simulink model "MFC_SISO"  (R2026a)
settings: Solver=VariableStepAuto  StopTime=t_simu
values from neighbouring files (symbols this model uses):
  a = 2.5348    [slexAircraftPitchControlData.mat]
  b = 64.13    [slexAircraftPitchControlData.mat]
  Md = -6.8847    [slexAircraftPitchControlData.mat]
  Mq = -0.6571    [slexAircraftPitchControlData.mat]
  Mw = -0.00592    [slexAircraftPitchControlData.mat]
  Swg = 3    [slexAircraftPitchControlData.mat]
  Uo = 689.4    [slexAircraftPitchControlData.mat]
  Vto = 690.4    [slexAircraftPitchControlData.mat]
  Zd = -63.9979    [slexAircraftPitchControlData.mat]
  Zw = -0.6385    [slexAircraftPitchControlData.mat]
undefined symbols (not defined in the file or in its folder): Ts
libraries: aerolibactuator x2, simulink x1
settings Model: Creator=devinbellll  LastModifiedBy=devinbellll

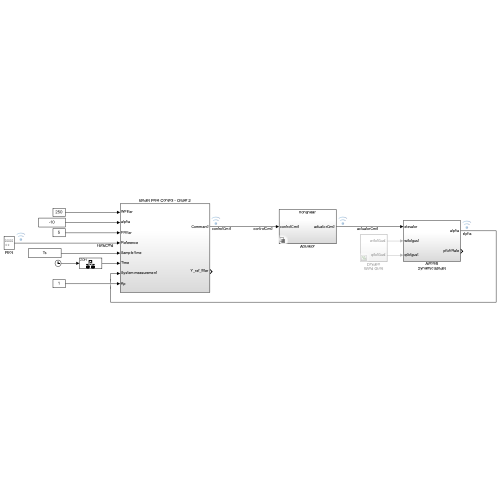
[thumbnail: Simulink's stored preview of the top-level diagram]
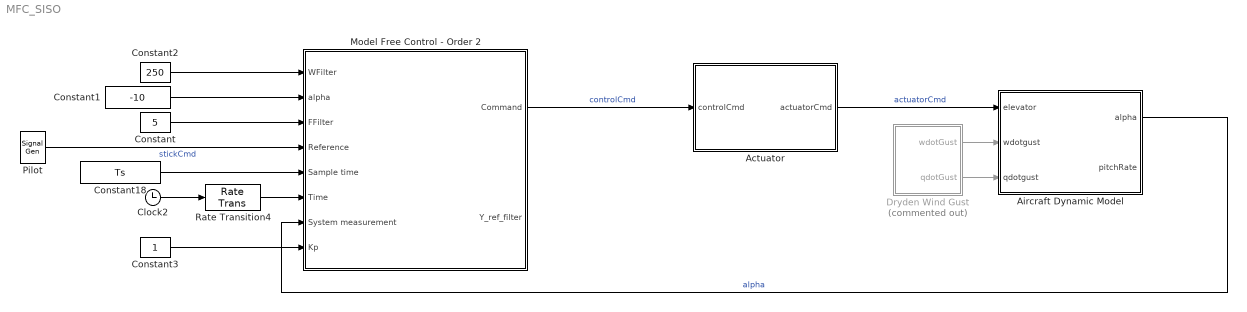
== system MFC_SISO ==
  Actuator : Subsystem  Variant=on  VariantControlMode=label  LabelModeActiveChoice=NonlinearActuator
  Aircraft Dynamic Model : Subsystem
  Clock2 : Clock
  Constant : Constant  Value=5
  Constant1 : Constant  Value=-10
  Constant18 : Constant  Value=Ts  SampleTime=-1
  Constant2 : Constant  Value=250
  Constant3 : Constant
  Dryden Wind Gust : Subsystem  Commented=on
  Model Free Control - Order 2 : Subsystem
  Pilot : SignalGenerator  WaveForm=square  Frequency=.1
  Rate Transition4 : RateTransition  OutPortSampleTime=Ts
  wires:
  Constant3/1 -> Model Free Control - Order 2/8(Kp)
  Clock2/1 -> Rate Transition4/1
  Rate Transition4/1 -> Model Free Control - Order 2/6(Time)
  Constant18/1 -> Model Free Control - Order 2/5(Sample time)
  Constant/1 -> Model Free Control - Order 2/3(FFilter)
  Pilot/1 -> Model Free Control - Order 2/4(Reference)  "stickCmd"
  Constant2/1 -> Model Free Control - Order 2/1(WFilter)
  Constant1/1 -> Model Free Control - Order 2/2(alpha)
  Model Free Control - Order 2/1(Command) -> Actuator/1(controlCmd)  "controlCmd"
  Dryden Wind Gust/1(wdotGust) -> Aircraft Dynamic Model/2(wdotgust)
  Actuator/1(actuatorCmd) -> Aircraft Dynamic Model/1(elevator)  "actuatorCmd"
  Dryden Wind Gust/2(qdotGust) -> Aircraft Dynamic Model/3(qdotgust)
  Aircraft Dynamic Model/1(alpha) -> Model Free Control - Order 2/7(System measurement)  "alpha"

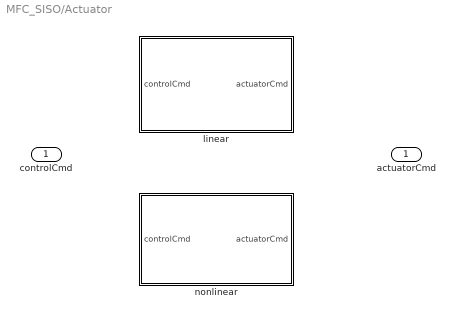
== system MFC_SISO/Actuator ==
  controlCmd : Inport
  linear : Subsystem  VariantControl=LinearActuator
  nonlinear : Subsystem  VariantControl=NonlinearActuator
  actuatorCmd : Outport  InitialOutput=0  VectorParamsAs1DForOutWhenUnconnected=off

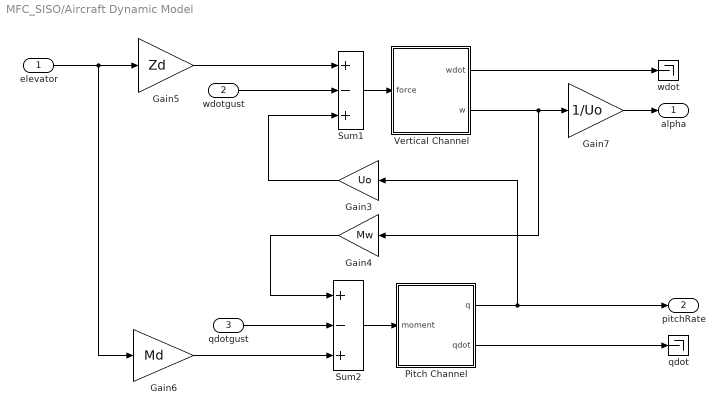
== system MFC_SISO/Aircraft Dynamic Model ==
  elevator : Inport
  wdotgust : Inport  Port=2
  qdotgust : Inport  Port=3
  Gain3 : Gain  Gain=Uo  SaturateOnIntegerOverflow=on  OutDataTypeStr=Inherit: Same as input  ParamDataTypeStr=Inherit: Same as input
  Gain4 : Gain  Gain=Mw  SaturateOnIntegerOverflow=on  OutDataTypeStr=Inherit: Same as input  ParamDataTypeStr=Inherit: Same as input
  Gain5 : Gain  Gain=Zd  SaturateOnIntegerOverflow=on  OutDataTypeStr=Inherit: Same as input  ParamDataTypeStr=Inherit: Same as input
  Gain6 : Gain  Gain=Md  SaturateOnIntegerOverflow=on  OutDataTypeStr=Inherit: Same as input  ParamDataTypeStr=Inherit: Same as input
  Gain7 : Gain  Gain=1/Uo  SaturateOnIntegerOverflow=on  OutDataTypeStr=Inherit: Same as input  ParamDataTypeStr=Inherit: Same as input
  Pitch Channel : Subsystem
  Sum1 : Sum  Inputs=+-+  InputSameDT=on  SaturateOnIntegerOverflow=on  OutDataTypeStr=Inherit: Same as first input
  Sum2 : Sum  Inputs=+-+  InputSameDT=on  SaturateOnIntegerOverflow=on  OutDataTypeStr=Inherit: Same as first input
  Vertical Channel : Subsystem
  qdot : Terminator
  wdot : Terminator
  alpha : Outport
  pitchRate : Outport  Port=2
  wires:
  Pitch Channel/1(q) -> Gain3/1, pitchRate/1
  Vertical Channel/2(w) -> Gain7/1, Gain4/1
  Sum1/1 -> Vertical Channel/1(force)
  Gain6/1 -> Sum2/3
  Gain5/1 -> Sum1/1
  qdotgust/1 -> Sum2/2
  Sum2/1 -> Pitch Channel/1(moment)
  wdotgust/1 -> Sum1/2
  elevator/1 -> Gain6/1, Gain5/1
  Gain7/1 -> alpha/1
  Gain3/1 -> Sum1/3
  Gain4/1 -> Sum2/1
  Vertical Channel/1(wdot) -> wdot/1
  Pitch Channel/2(qdot) -> qdot/1

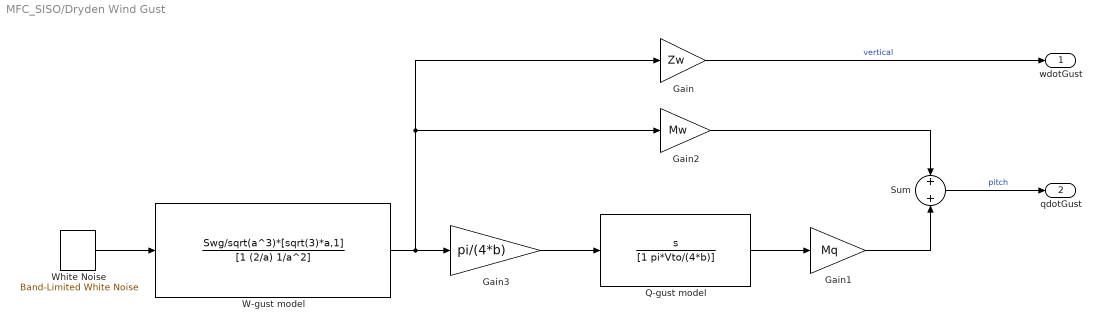
== system MFC_SISO/Dryden Wind Gust ==
  Gain : Gain  Gain=Zw  SaturateOnIntegerOverflow=on  OutDataTypeStr=Inherit: Same as input  ParamDataTypeStr=Inherit: Same as input
  Gain1 : Gain  Gain=Mq  SaturateOnIntegerOverflow=on  OutDataTypeStr=Inherit: Same as input  ParamDataTypeStr=Inherit: Same as input
  Gain2 : Gain  Gain=Mw  SaturateOnIntegerOverflow=on  OutDataTypeStr=Inherit: Same as input  ParamDataTypeStr=Inherit: Same as input
  Gain3 : Gain  Gain=pi/(4*b)  SaturateOnIntegerOverflow=on  OutDataTypeStr=Inherit: Same as input  ParamDataTypeStr=Inherit: Same as input
  Q-gust model : TransferFcn  Numerator=[1 0]  Denominator=[1 pi*Vto/(4*b)]
  Sum : Sum  InputSameDT=on  SaturateOnIntegerOverflow=on  OutDataTypeStr=Inherit: Same as first input
  W-gust model : TransferFcn  Numerator=Swg/sqrt(a^3)*[sqrt(3)*a,1]  Denominator=[1 (2/a) 1/a^2]
  White Noise : simulink/Sources/Band-Limited White Noise  Cov=10  Ts=0.01  seed=23341
  wdotGust : Outport  VectorParamsAs1DForOutWhenUnconnected=off
  qdotGust : Outport  Port=2  VectorParamsAs1DForOutWhenUnconnected=off
  wires:
  Gain/1 -> wdotGust/1  "vertical"
  White Noise/1 -> W-gust model/1
  Gain3/1 -> Q-gust model/1
  Sum/1 -> qdotGust/1  "pitch"
  Gain2/1 -> Sum/1
  Q-gust model/1 -> Gain1/1
  W-gust model/1 -> Gain/1, Gain2/1, Gain3/1
  Gain1/1 -> Sum/2

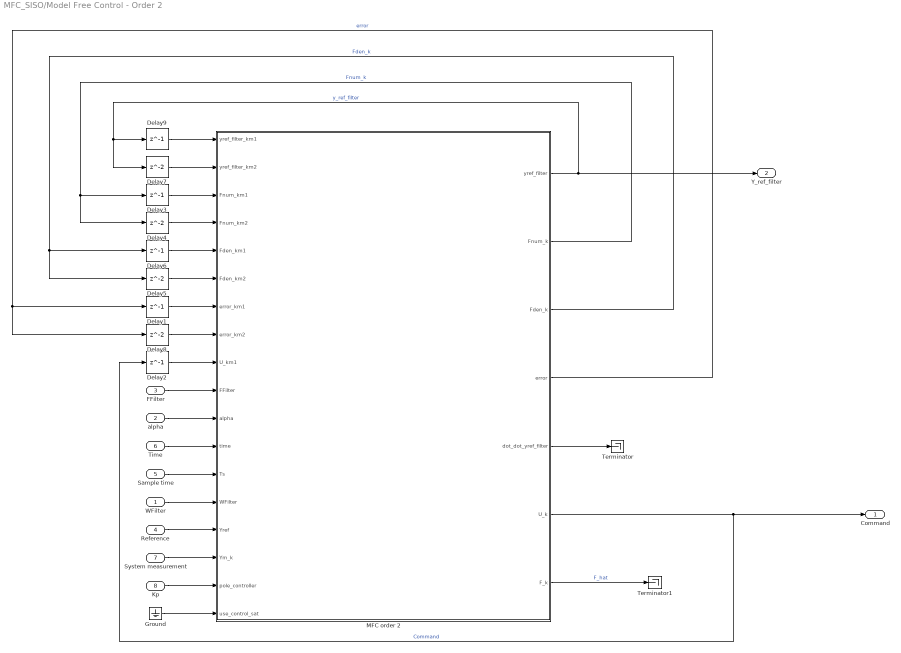
== system MFC_SISO/Model Free Control - Order 2 ==
  WFilter : Inport
  alpha : Inport  Port=2
  FFilter : Inport  Port=3
  Reference : Inport  Port=4
  Sample time : Inport  Port=5
  Time : Inport  Port=6
  System measurement : Inport  Port=7
  Kp : Inport  Port=8
  Delay{1..3,6} (4 alike) : Delay  DelayLength=1  SampleTime=Ts
  Delay4 : Delay  SampleTime=Ts
  Delay5 : Delay  SampleTime=Ts
  Delay7 : Delay  InitialCondition=0  SampleTime=Ts
  Delay8 : Delay  SampleTime=Ts
  Delay9 : Delay  DelayLength=1  InitialCondition=0  SampleTime=Ts
  Ground : Ground
  MFC order 2 : MATLAB Function  Tag=ULM  TreatAsAtomicUnit=on
  Terminator : Terminator
  Terminator1 : Terminator
  Command : Outport  VectorParamsAs1DForOutWhenUnconnected=off
  Y_ref_filter : Outport  Port=2  VectorParamsAs1DForOutWhenUnconnected=off
  wires:
  MFC order 2/5(dot_dot_yref_filter) -> Terminator/1
  Ground/1 -> MFC order 2/18(use_control_sat)
  MFC order 2/7(F_k) -> Terminator1/1  "F_hat"
  Reference/1 -> MFC order 2/15(Yref)
  MFC order 2/4(error) -> Delay1/1, Delay8/1  "error"
  MFC order 2/1(yref_filter) -> Delay9/1, Delay7/1, Y_ref_filter/1  "y_ref_filter"
  Kp/1 -> MFC order 2/17(pole_controller)
  MFC order 2/3(Fden_k) -> Delay5/1, Delay6/1  "Fden_k"
  MFC order 2/2(Fnum_k) -> Delay3/1, Delay4/1  "Fnum_k"
  Delay7/1 -> MFC order 2/2(yref_filter_km2)
  Delay9/1 -> MFC order 2/1(yref_filter_km1)
  MFC order 2/6(U_k) -> Delay2/1, Command/1  "Command"
  Delay8/1 -> MFC order 2/8(error_km2)
  Delay1/1 -> MFC order 2/7(error_km1)
  WFilter/1 -> MFC order 2/14(WFilter)
  System measurement/1 -> MFC order 2/16(Ym_k)
  alpha/1 -> MFC order 2/11(alpha)
  FFilter/1 -> MFC order 2/10(FFilter)
  Sample time/1 -> MFC order 2/13(Ts)
  Time/1 -> MFC order 2/12(time)
  Delay5/1 -> MFC order 2/6(Fden_km2)
  Delay3/1 -> MFC order 2/3(Fnum_km1)
  Delay6/1 -> MFC order 2/5(Fden_km1)
  Delay4/1 -> MFC order 2/4(Fnum_km2)
  Delay2/1 -> MFC order 2/9(U_km1)

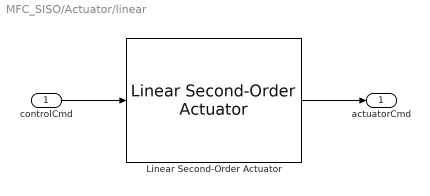
== system MFC_SISO/Actuator/linear ==
  controlCmd : Inport
  Linear Second-Order Actuator : aerolibactuator/Linear Second-Order Actuator  wn_fin=44.721  z_fin=1.118  fin_act_0=0  fin_act_vel=0
  actuatorCmd : Outport  InitialOutput=0  VectorParamsAs1DForOutWhenUnconnected=off
  wires:
  controlCmd/1 -> Linear Second-Order Actuator/1
  Linear Second-Order Actuator/1 -> actuatorCmd/1

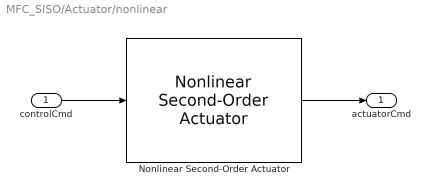
== system MFC_SISO/Actuator/nonlinear ==
  controlCmd : Inport
  Nonlinear Second-Order Actuator : aerolibactuator/Nonlinear Second-Order Actuator  wn_fin=44.721  z_fin=1.118  fin_max=45*pi/180  fin_min=-45*pi/180  fin_maxrate=500*pi/180  fin_act_0=0  fin_act_vel=0
  actuatorCmd : Outport  InitialOutput=0  VectorParamsAs1DForOutWhenUnconnected=off
  wires:
  controlCmd/1 -> Nonlinear Second-Order Actuator/1
  Nonlinear Second-Order Actuator/1 -> actuatorCmd/1

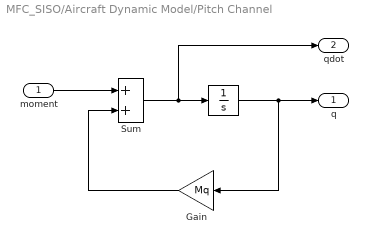
== system MFC_SISO/Aircraft Dynamic Model/Pitch Channel ==
  moment : Inport
  " " : Integrator
  Gain : Gain  Gain=Mq  SaturateOnIntegerOverflow=on  OutDataTypeStr=Inherit: Same as input  ParamDataTypeStr=Inherit: Same as input
  Sum : Sum  InputSameDT=on  SaturateOnIntegerOverflow=on  OutDataTypeStr=Inherit: Same as first input
  q : Outport
  qdot : Outport  Port=2
  wires:
  moment/1 -> Sum/1
  Gain/1 -> Sum/2
  " "/1 -> q/1, Gain/1
  Sum/1 -> qdot/1, " "/1

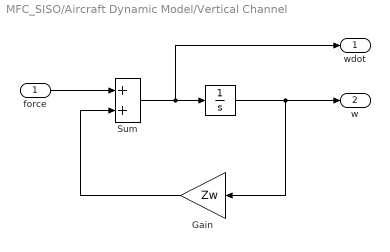
== system MFC_SISO/Aircraft Dynamic Model/Vertical Channel ==
  force : Inport
  " " : Integrator
  Gain : Gain  Gain=Zw  SaturateOnIntegerOverflow=on  OutDataTypeStr=Inherit: Same as input  ParamDataTypeStr=Inherit: Same as input
  Sum : Sum  InputSameDT=on  SaturateOnIntegerOverflow=on  OutDataTypeStr=Inherit: Same as first input
  wdot : Outport
  w : Outport  Port=2
  wires:
  Sum/1 -> wdot/1, " "/1
  " "/1 -> w/1, Gain/1
  Gain/1 -> Sum/2
  force/1 -> Sum/1

== matlab function MFC_SISO/Model Free Control - Order 2/MFC order 2 ==
  data: yref_filter_km1 input; yref_filter_km2 input; Fnum_km1 input; Fnum_km2 input; Fden_km1 input; Fden_km2 input; error_km1 input; error_km2 input; U_km1 input; yref_filter output; FFilter input; alpha input; time input; Ts input; WFilter input; Yref input; Ym_k input; Fnum_k output; Fden_k output; error output; dot_dot_yref_filter output; U_k output; pole_controller input; F_k output; use_control_sat input
function [yref_filter, Fnum_k, Fden_k, error, dot_dot_yref_filter, U_k, F_k] = MFC_order2(yref_filter_km1, yref_filter_km2, Fnum_km1, Fnum_km2, Fden_km1, Fden_km2, error_km1, error_km2, U_km1, FFilter, alpha, time, Ts, WFilter, Yref, Ym_k, pole_controller, use_control_sat)
    
% 1) Referene filter
    yref_filter = (Yref + (2*WFilter^2+2*WFilter)*yref_filter_km1+(-WFilter^2)*yref_filter_km2)/(WFilter^2+2*WFilter+1);
    %yref_filter = 90*(pi/180) + yref_filter;
    %yref_filter = Y;
    dot_yref_filter     = (yref_filter-yref_filter_km1)/Ts;
    dot_dot_yref_filter = (yref_filter-2*yref_filter_km1+yref_filter_km2)/(Ts^2);
    
% 2) Control poles (s-p)^2=s^2+as+b
    a = -2*pole_controller;
    b = -pole_controller^2;
       
    % With error
    error = Ym_k - yref_filter;
    
    % ddoty = F+alpha*u+a.dote+b.e
    sde   = -(time*error-(time-Ts)*error_km1)/Ts;
    s2d2e =  (time^2*error-2*(time-Ts)^2*error_km1+(time-2*Ts)^2*error_km2)/(Ts^2);
    sd2e  =  (time^2*error-(time-Ts)^2*error_km1)/Ts;
    de    = -time*error;
    d2e   =  time^2*error;
    d2u   =  time^2*U_km1;
    
    % d^2/ds^2 ->
    num = 2*error+4*sde+s2d2e-a*(2*de+sd2e)-b*(d2e)-alpha*d2u;  
    den = time^2;
    
% 3) Filter and estimator F    
    Fnum_k = (num+(2*FFilter^2+2*FFilter)*Fnum_km1+(-FFilter^2)*Fnum_km2)/(FFilter^2+2*FFilter+1);
    Fden_k = (den+(2*FFilter^2+2*FFilter)*Fden_km1+(-FFilter^2)*Fden_km2)/(FFilter^2+2*FFilter+1);
    
    F_k=0; 
    if (Fden_k~=0)&&(time>.1)%0.1
        F_k=Fnum_k/Fden_k;
    end

%% Command generation
    U_k = -F_k/alpha + dot_dot_yref_filter/alpha;

% Saturation
if(use_control_sat)
     U_k = max(-600, U_k);
     U_k = min(600,  U_k);
end
UFilter = 1;

%Filter of U eventually necessary
    U_k = (U_k+(UFilter-1)*U_km1)/UFilter;
